simulink model "operational_space_pd_w_g_comp"  (R2020b)
settings: Solver=VariableStepAuto  StartTime=0.0  StopTime=10.0  RelTol=1e-3
undefined symbols (not defined in the file): dqi, g_q, KD, KP, myRobot, qi, Ts, xf
libraries: vrlib x1
settings Model: Creator=simon  LastModifiedBy=SimoneCremasco

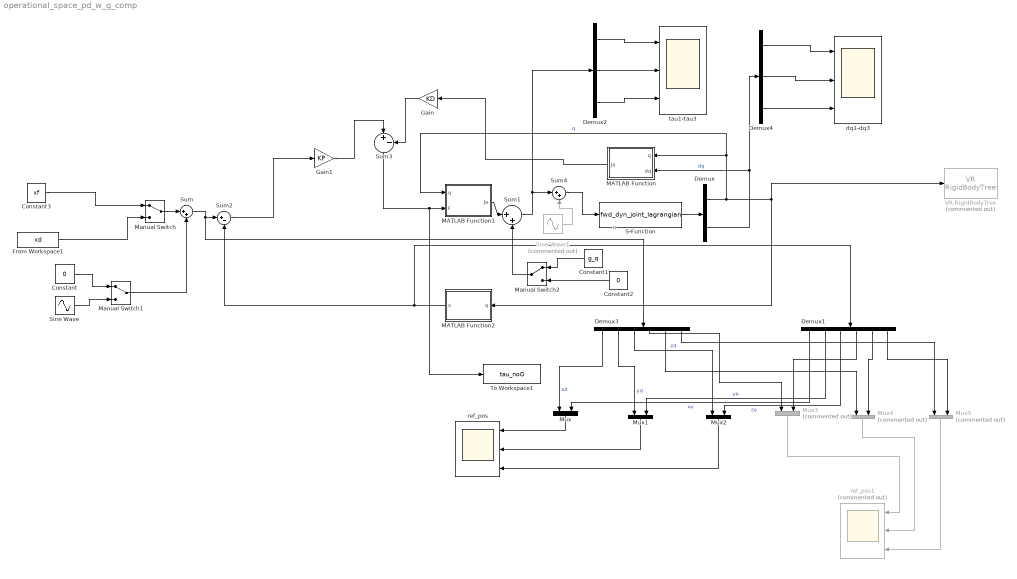
== system operational_space_pd_w_g_comp ==
  note: u
  Constant : Constant  Value=0
  Constant1 : Constant  Value=g_q
  Constant2 : Constant  Value=0
  Constant3 : Constant  Value=xf
  Demux : Demux  Outputs=2
  Demux1 : Demux  Outputs=6
  Demux2 : Demux  Outputs=myRobot.N
  Demux3 : Demux  Outputs=6
  Demux4 : Demux  Outputs=myRobot.N
  From Workspace1 : FromWorkspace  VariableName=xd  SampleTime=Ts
  Gain : Gain  Gain=KD
  Gain1 : Gain  Gain=KP
  MATLAB Function : MATLAB Function  TreatAsAtomicUnit=on
  MATLAB Function1 : MATLAB Function  TreatAsAtomicUnit=on
  MATLAB Function2 : MATLAB Function  TreatAsAtomicUnit=on
  Manual Switch : ManualSwitch
  Manual Switch1 : ManualSwitch
  Manual Switch2 : ManualSwitch
  Mux : Mux  Inputs=2
  Mux1 : Mux  Inputs=2
  Mux2 : Mux  Inputs=2
  Mux3 : Mux  Commented=on  Inputs=2
  Mux4 : Mux  Commented=on  Inputs=2
  Mux5 : Mux  Commented=on  Inputs=2
  S-Function : S-Function  FunctionName=fwd_dyn_joint_lagrangian  Parameters=myRobot,qi,dqi  SFunctionDeploymentMode=off  EnableBusSupport=off
  Sine Wave : Sin  Amplitude=0.1  SampleTime=0
  Sine Wave1 : Sin  Commented=on  Amplitude=0.1  Frequency=5  SampleTime=0
  Sum : Sum  Inputs=|++
  Sum1 : Sum  Inputs=|++
  Sum2 : Sum  Inputs=|+-
  Sum3 : Sum  Inputs=|+-
  Sum4 : Sum  Inputs=|++
  To Workspace1 : ToWorkspace  VariableName=tau_noG  SaveFormat=Timeseries  SampleTime=-1
  VR RigidBodyTree : vrlib/VR RigidBodyTree  Commented=on  RBT=rbt  useRBT=on  Ts=-1  ForceViewerOpen=on
      settings: SourceProductBaseCode=SL
  dq1-dq3 : Scope  NumInputPorts=3
  ref_pos : Scope  NumInputPorts=3
  ref_pos1 : Scope  Commented=on  NumInputPorts=3
  tau1-tau3 : Scope  NumInputPorts=3
  wires:
  Constant1/1 -> Manual Switch2/1
  Constant2/1 -> Manual Switch2/2
  Constant/1 -> Manual Switch1/1
  Mux2/1 -> ref_pos/3
  Manual Switch1/1 -> Sum/2
  Demux3/2 -> Mux1/1  "yd"
  Sine Wave1/1 -> Sum4/2
  Mux1/1 -> ref_pos/2
  Demux3/1 -> Mux/1  "xd"
  Mux/1 -> ref_pos/1
  Manual Switch/1 -> Sum/1
  Sum4/1 -> S-Function/1
  From Workspace1/1 -> Manual Switch/2
  Demux2/3 -> tau1-tau3/3
  Sum/1 -> Demux3/1, Sum2/1
  Manual Switch2/1 -> Sum1/2
  Sum1/1 -> Sum4/1, Demux2/1
  Demux1/3 -> Mux2/2  "ze"
  Demux4/1 -> dq1-dq3/1
  Demux4/3 -> dq1-dq3/3
  Constant3/1 -> Manual Switch/1
  Demux/1 -> MATLAB Function1/1(q), MATLAB Function/1(q), VR RigidBodyTree/1, MATLAB Function2/1(q)  "q"
  Sum2/1 -> Gain1/1
  Demux4/2 -> dq1-dq3/2
  Sine Wave/1 -> Manual Switch1/2
  Gain1/1 -> Sum3/1
  Demux1/1 -> Mux/2  "xe"
  Sum3/1 -> To Workspace1/1, MATLAB Function1/2(F)
  Demux3/3 -> Mux2/1  "zd"
  S-Function/1 -> Demux/1
  Demux/2 -> MATLAB Function/2(dq), Demux4/1  "dq"
  Gain/1 -> Sum3/2
  Demux1/2 -> Mux1/2  "ye"
  Demux2/1 -> tau1-tau3/1
  Demux2/2 -> tau1-tau3/2
  MATLAB Function/1(Ja) -> Gain/1
  MATLAB Function1/1(Ja) -> Sum1/1
  MATLAB Function2/1(x) -> Sum2/2, Demux1/1
  Demux1/5 -> Mux4/2
  Demux3/4 -> Mux3/1
  Demux3/5 -> Mux4/1
  Demux1/6 -> Mux5/2
  Demux1/4 -> Mux3/2
  Demux3/6 -> Mux5/1
  Mux3/1 -> ref_pos1/1
  Mux4/1 -> ref_pos1/2
  Mux5/1 -> ref_pos1/3

== matlab function operational_space_pd_w_g_comp/MATLAB Function ==
  data: q input size=3; Ja output; dq input
function Ja = fcn(q, dq)

Ja = getJa(q)*dq;

== matlab function operational_space_pd_w_g_comp/MATLAB Function2 ==
  data: q input; x output
function x = fcn(q)
x = getK(q);

== matlab function operational_space_pd_w_g_comp/MATLAB Function1 ==
  data: q input size=3; Ja output size=3; F input
function Ja = fcn(q, F)

Ja = getJa(q)'*F;
